simulink model "MagLevTbx_MagSens_Block"  (R2025b)
settings: Solver=VariableStepAuto  StartTime=0.0  StopTime=10.0  RelTol=1e-3
settings Model: Creator=riccardo  LastModifiedBy=riccardo

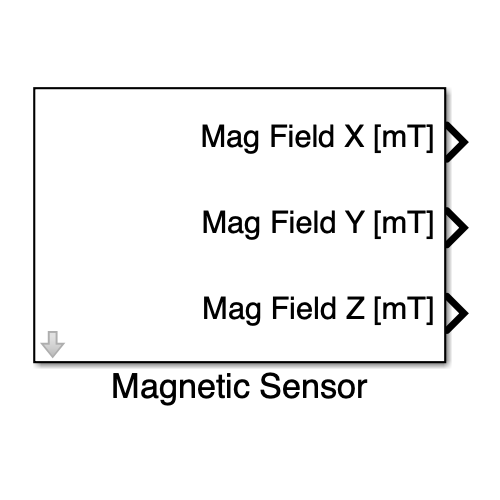
[thumbnail: Simulink's stored preview of the top-level diagram]
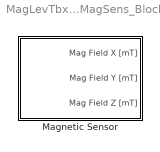
== system MagLevTbx_MagSens_Block ==
  Magnetic Sensor : Subsystem  mask(Magnetic Sensor (Infineon TLV493D)){sensorId=Sensor 7, sampleTime=-1, showEnablePort=off}
      mask prompts: sensorId "Magnetic Sensor:"; sampleTime "Sample time (-1 for inherited):"; showEnablePort "Show enable port"
      mask help: Get 3D magnetic field measurement (in [mT]) from the selected magnetic sensor.
      mask init:
      | %   select block variant according to hardware (PCB) version
      | blk = gcb;
      | vss = [blk '/MagSens'];
      | 
      | m = Simulink.Mask.get(gcb);
      | pSensorId = m.getParameter('sensorId');
      | 
      | group = "MagLevTbx";
      | pref  = "HwVersion";
      | 
      | if ispref(group, pref)
      |     hwVer = getpref(group, pref);
      |     switch hwVer 
      |         case '4.0'
      |             set_param(vss, 'LabelModeActiveChoice', '4.0');
      |             pSensorId.Visible = 'on';
      |         case '4.3'
      |             set_param(vss, 'LabelModeActiveChoice', '4.3');
      |             pSensorId.Visible = 'off';
      |         otherwise
      |             error('Unsupported PCB version: %s', hwVer);
      |     end
      | else
      |     hwVer = 0;
      |     disp('ciao')
      |     error('MagLevTbx:PCBVersionNotConfigured', ...
      |         'MagLev PCB version not configured. Please run MagLevTbx_HwConfig() to set the hardware version.');
      | end
      | 
      | %   add/remove enable block
      | MagLevTbx_MagSens_MaskInit(gcb, showEnablePort);
      mask Help:
      | Riccardo Antonello (riccardo.antonello@unipd.it)
      | 
      | February 17, 2026
      | 
      | Dept. of Information Engineering, University of Padova
      mask Callback sampleTime: MagLevTbx_MagSens_MaskCbFcn_SampleTime();

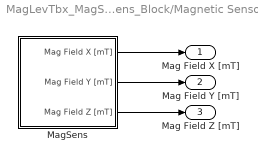
== system MagLevTbx_MagSens_Block/Magnetic Sensor ==
  MagSens : Subsystem  Variant=on  VariantControlMode=label  LabelModeActiveChoice=4.0
  Mag Field X [mT] : Outport
  Mag Field Y [mT] : Outport  Port=2
  Mag Field Z [mT] : Outport  Port=3
  wires:
  MagSens/1(Mag Field X [mT]) -> Mag Field X [mT]/1
  MagSens/2(Mag Field Y [mT]) -> Mag Field Y [mT]/1
  MagSens/3(Mag Field Z [mT]) -> Mag Field Z [mT]/1

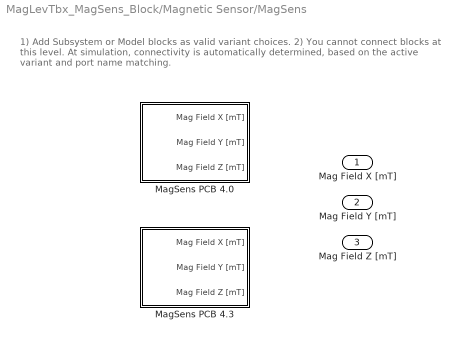
== system MagLevTbx_MagSens_Block/Magnetic Sensor/MagSens ==
  note: 1) Add Subsystem or Model blocks as valid variant choices.
      | 2) You cannot connect blocks at this level. At simulation, connectivity is automatically
      | determined, based on the active variant and port name matching.
  MagSens PCB 4.0 : Subsystem  VariantControl=4.0
  MagSens PCB 4.3 : Subsystem  VariantControl=4.3
  Mag Field X [mT] : Outport
  Mag Field Y [mT] : Outport  Port=2
  Mag Field Z [mT] : Outport  Port=3

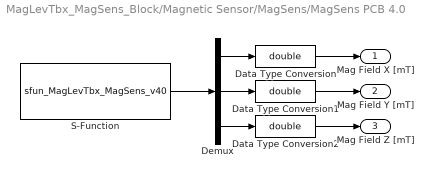
== system MagLevTbx_MagSens_Block/Magnetic Sensor/MagSens/MagSens PCB 4.0 ==
  Data Type Conversion : DataTypeConversion  OutDataTypeStr=double  SaturateOnIntegerOverflow=off  RndMeth=Floor
  Data Type Conversion1 : DataTypeConversion  OutDataTypeStr=double  SaturateOnIntegerOverflow=off  RndMeth=Floor
  Data Type Conversion2 : DataTypeConversion  OutDataTypeStr=double  SaturateOnIntegerOverflow=off  RndMeth=Floor
  Demux : Demux  Outputs=3
  S-Function : S-Function  FunctionName=sfun_MagLevTbx_MagSens_v40  Parameters=sensorId, sampleTime  SFunctionDeploymentMode=off  EnableBusSupport=off
  Mag Field X [mT] : Outport
  Mag Field Y [mT] : Outport  Port=2
  Mag Field Z [mT] : Outport  Port=3
  wires:
  Data Type Conversion1/1 -> Mag Field Y [mT]/1
  Demux/2 -> Data Type Conversion1/1
  Demux/3 -> Data Type Conversion2/1
  Data Type Conversion/1 -> Mag Field X [mT]/1
  S-Function/1 -> Demux/1
  Demux/1 -> Data Type Conversion/1
  Data Type Conversion2/1 -> Mag Field Z [mT]/1

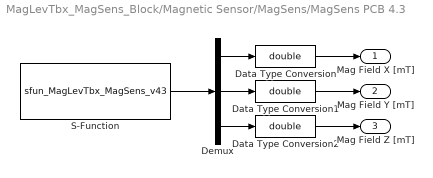
== system MagLevTbx_MagSens_Block/Magnetic Sensor/MagSens/MagSens PCB 4.3 ==
  Data Type Conversion : DataTypeConversion  OutDataTypeStr=double  SaturateOnIntegerOverflow=off  RndMeth=Floor
  Data Type Conversion1 : DataTypeConversion  OutDataTypeStr=double  SaturateOnIntegerOverflow=off  RndMeth=Floor
  Data Type Conversion2 : DataTypeConversion  OutDataTypeStr=double  SaturateOnIntegerOverflow=off  RndMeth=Floor
  Demux : Demux  Outputs=3
  S-Function : S-Function  FunctionName=sfun_MagLevTbx_MagSens_v43  Parameters=sampleTime  SFunctionDeploymentMode=off  EnableBusSupport=off
  Mag Field X [mT] : Outport
  Mag Field Y [mT] : Outport  Port=2
  Mag Field Z [mT] : Outport  Port=3
  wires:
  Data Type Conversion2/1 -> Mag Field Z [mT]/1
  Demux/1 -> Data Type Conversion/1
  S-Function/1 -> Demux/1
  Data Type Conversion/1 -> Mag Field X [mT]/1
  Demux/3 -> Data Type Conversion2/1
  Demux/2 -> Data Type Conversion1/1
  Data Type Conversion1/1 -> Mag Field Y [mT]/1
